simulink model "untitled"  (R2021b)
settings: Solver=FixedStepDiscrete  StartTime=0.0  StopTime=10.0  FixedStep=0.2  RelTol=1e-3
undefined symbols (not defined in the file): sldvsubsys
libraries: simulink x2, sldvlib x1
settings Model: Creator=Alessandro  LastModifiedBy=Alessandro
settings ConfigComp: DVMode=PropertyProving  DVTestSuiteOptimization=Auto  DVDetectOutOfBounds=on  DVModelReferenceHarness=on

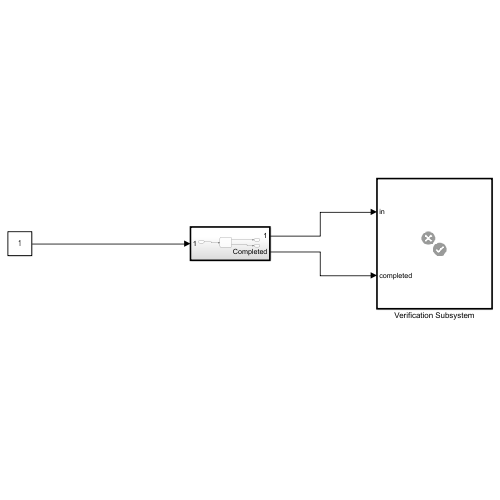
[thumbnail: Simulink's stored preview of the top-level diagram]
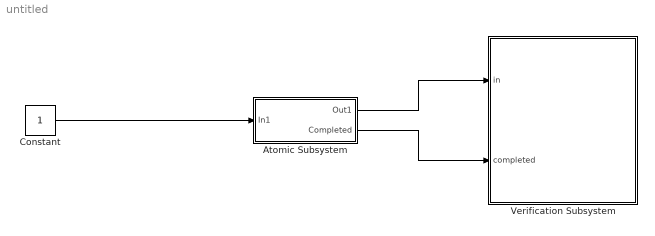
== system untitled ==
  Atomic Subsystem : Subsystem  TreatAsAtomicUnit=on
  Constant : Constant  VectorParams1D=off
  Verification Subsystem : Subsystem  Tag=VerificationSubsystem  DisableCoverage=on  LoadFcn=sldvsubsys('check')  TreatAsAtomicUnit=on  SimViewingDevice=on  mask(VerificationSubsystem){}
      mask init:
      | sldvsubsys('maskInit');
      settings: CopyFcn=sldvsubsys('copy');  OpenFcn=open_system(gcb,'force');
      settings: PreSaveFcn=|
      | set_param(gcb,'SimViewingDevice','on');
      | sldvsubsys('check');
      mask Help: helpview(fullfile(docroot,'toolbox','sldv','sldv.map'),'verificationsubsystem')
      mask Display: image(imread('sldvicon_versubsys.png','BackGroundColor',[1 1 1]),'center');
  wires:
  Constant/1 -> Atomic Subsystem/1(In1)
  Atomic Subsystem/1(Out1) -> Verification Subsystem/1(in)
  Atomic Subsystem/2(Completed) -> Verification Subsystem/2(completed)

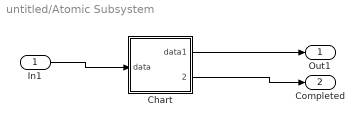
== system untitled/Atomic Subsystem ==
  In1 : Inport
  Chart : Stateflow chart  TreatAsAtomicUnit=on
  Out1 : Outport
  Completed : Outport  Port=2
  wires:
  In1/1 -> Chart/1(data)
  Chart/1(data1) -> Out1/1
  Chart/2(completed) -> Completed/1

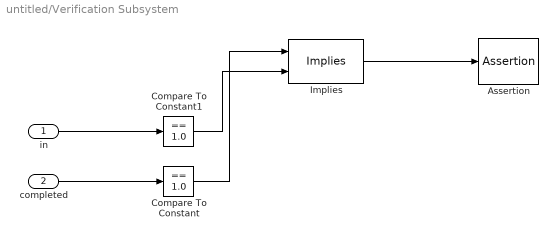
== system untitled/Verification Subsystem ==
  in : Inport
  completed : Inport  Port=2
  Assertion : Assertion  StopWhenAssertionFail=off
  Compare To Constant : simulink/Logic and Bit Operations/Compare To Constant  relop===  const=1.0  OutDataTypeStr=boolean
  Compare To Constant1 : simulink/Logic and Bit Operations/Compare To Constant  relop===  const=1.0  OutDataTypeStr=boolean
  Implies : sldvlib/Verification Utilities/Implies
      settings: SourceProductBaseCode=SL
  wires:
  completed/1 -> Compare To Constant/1
  in/1 -> Compare To Constant1/1
  Compare To Constant/1 -> Implies/1
  Compare To Constant1/1 -> Implies/2
  Implies/1 -> Assertion/1

== stateflow chart untitled/Atomic Subsystem/Chart ==
  state begin
  state Stato1
    entry:
    data1 = data;
    completed = 1;
  (default) -> begin
  begin -> Stato1 : [data>0]
  data: data input; data1 output; completed output
